simulink model "ECO_openSource"  (R2020b)
settings: Solver=FixedStepAuto  StartTime=0.0  StopTime=parECO.ref.time(end)+parECO.ref.dT  FixedStep=0.001  RelTol=1e-3  EnableMultiTasking=on
InitFcn:
  | if ~exist('parECO','var')
  |    load('parECO.mat');
  | end
  | if ~isfield(parECO,'ref')
  | 
  |    parECO.enNoise = true;
  |    parECO.enDist = true;
  |    parECO.enFB.imep = true;
  |    parECO.enFB.dpMax = true;
  |    parECO.enFB.Tevo = true;
  |    parECO.enFB.cNOx = true;
  | 
  |    parECO.ref.dT = 5;
  |    parECO.ref.imep = [  6   6   9   9   7   7 ] * 1e5
  |    parECO.ref.dpMax = [ 15   4   4   4   4   4 ] * 1e5;
  |    parECO.ref.Tevo = [  0   0   0 680   0   0 ] + 273;
  |    parECO.ref.cNOx = [100 100 100 100 100  15 ] * 1e2;
  | 
  |    parECO.ref.time  = 0 : parECO.ref.dT : parECO.ref.dT*(numel(parECO.ref.imep)-1);
  |    parECO.ref.imep  = [parECO.Reference.IMEP parECO.ref.imep(1)  parECO.ref.imep ];
  |    parECO.ref.dpMax = [parECO.Reference.dpMax parECO.ref.dpMax(1) parECO.ref.dpMax];
  |    parECO.ref.Tevo  = [parECO.Reference.Tmin parECO.ref.Tevo(1)  parECO.ref.Tevo];
  |    parECO.ref.cNOx  = [parECO.Reference.cNOx parECO.ref.cNOx(1)  parECO.ref.cNOx];
  |    parECO.ref.time  = [0 1 parECO.ref.time + parECO.ref.dT ];
  | 
  | end
undefined symbols (not defined in the file): DiscIntNeverNeededParam, parOpt, parSim
libraries: simulink x6, dspstat3 x4, dspswit3 x1, hdlsllib x1
(part 2 of 2)

== system ECO_openSource/Controller/NMPC Algorithm/Subsystem/Algorithm/Create Bounds on h_e/Scale Reference ==
  unscaled : Inport
  Sum : Sum  Inputs=|++
  offs : Constant  Value=[parECO.offsX(3); 0]
  scale : Gain  Gain=1./[parECO.scaleX(3); 1e3]
  scaled : Outport
  wires:
  unscaled/1 -> scale/1
  scale/1 -> Sum/1
  Sum/1 -> scaled/1
  offs/1 -> Sum/2

== system ECO_openSource/Controller/NMPC Algorithm/Subsystem/Algorithm/Create Bounds on h_e/Scale cNOx ==
  unscaled : Inport
  Sum : Sum  Inputs=|++
  offs : Constant  Value=0
  scale : Gain  Gain=1./1e3
  scaled : Outport
  wires:
  unscaled/1 -> scale/1
  scale/1 -> Sum/1
  Sum/1 -> scaled/1
  offs/1 -> Sum/2

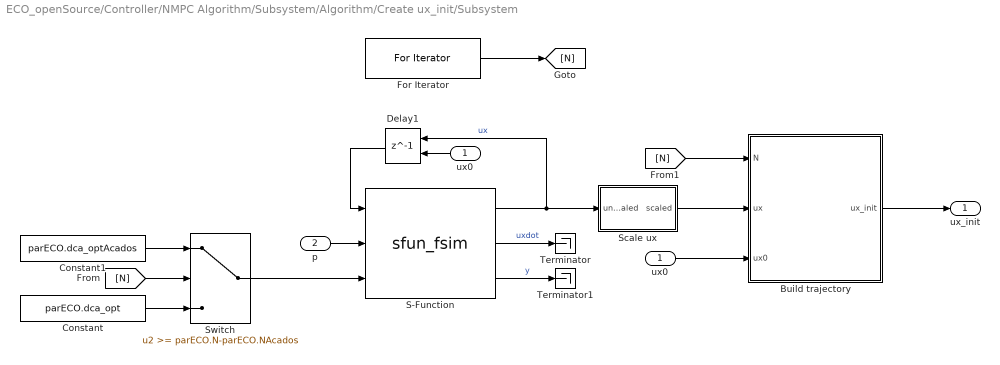
== system ECO_openSource/Controller/NMPC Algorithm/Subsystem/Algorithm/Create ux_init/Subsystem ==
  ux0 : Inport
  p : Inport  Port=2
  " ux0 " : InportShadow
  Build trajectory : Subsystem
  Constant : Constant  Value=parECO.dca_opt
  Constant1 : Constant  Value=parECO.dca_optAcados
  Delay1 : Delay  DelayLength=1  InitialConditionSource=Input port  InitialCondition=[parOpt.u0;parSim.OP.pInt;0;0]
      settings: InputPortMap=u0,p4
  For Iterator : ForIterator  ResetStates=reset  IterationLimit=parECO.N
  S-Function : S-Function  FunctionName=sfun_fsim  SFunctionDeploymentMode=off  EnableBusSupport=off
  Scale ux : Subsystem
  Switch : Switch  Threshold=parECO.N-parECO.NAcados
  Terminator : Terminator
  Terminator1 : Terminator
  ux_init : Outport
  wires:
  ux0/1 -> Delay1/2
  Delay1/1 -> S-Function/1
  " ux0 "/1 -> Build trajectory/3(ux0)
  Scale ux/1(scaled) -> Build trajectory/2(ux)
  Build trajectory/1(ux_init) -> ux_init/1
  Switch/1 -> S-Function/3
  Constant/1 -> Switch/3
  Constant1/1 -> Switch/1
  S-Function/1 -> Scale ux/1(unscaled), Delay1/1  "ux"
  S-Function/3 -> Terminator1/1  "y"
  S-Function/2 -> Terminator/1  "uxdot"
  For Iterator/1 -> [N]
  [N] -> Switch/2
  [N] -> Build trajectory/1(N)
  p/1 -> S-Function/2

== system ECO_openSource/Controller/NMPC Algorithm/Subsystem/Algorithm/Create ux_init/Unscale ux0 ==
  scaled : Inport
  Sum : Sum  Inputs=|++
  offs : Constant  Value=[parECO.offsU;parECO.offsX;parECO.offsCA]
  scale : Gain  Gain=[parECO.scaleU;parECO.scaleX;parECO.scaleCA]
  unscaled : Outport
  wires:
  offs/1 -> Sum/2
  scaled/1 -> scale/1
  scale/1 -> Sum/1
  Sum/1 -> unscaled/1

== system ECO_openSource/Controller/NMPC Algorithm/Subsystem/Algorithm/Model Simulation/Create Outputs ==
  ux : Inport
  uxdot : Inport  Port=2
  y : Inport  Port=3
  Delay : Delay  DelayLength=1
  Max : MinMax  Function=max  Inputs=2
  Mux : Mux
  Selector : Selector  InputPortWidth=10  IndexOptions=Index vector (dialog)  Indices=7  OutputSizes=1
  Selector1 : Selector  InputPortWidth=10  IndexOptions=Index vector (dialog)  Indices=5  OutputSizes=1
  Selector2 : Selector  InputPortWidth=12  IndexOptions=Index vector (dialog)  Indices=1  OutputSizes=1
  Selector3 : Selector  InputPortWidth=12  IndexOptions=Index vector (dialog)  Indices=9  OutputSizes=1
  ySim : Outport
  wires:
  ux/1 -> Selector/1
  uxdot/1 -> Selector1/1
  Selector1/1 -> Max/1
  Delay/1 -> Max/2
  Max/1 -> Delay/1, Mux/4
  Selector/1 -> Mux/1
  Mux/1 -> ySim/1
  Selector2/1 -> Mux/3
  Selector3/1 -> Mux/2
  y/1 -> Selector2/1, Selector3/1

== system ECO_openSource/Controller/NMPC Algorithm/Subsystem/Algorithm/Calculate Initial Condition/Calculate Condition at Start of Optimization/Scale ux0 ==
  unscaled : Inport
  Sum : Sum  Inputs=|+-
  offs : Constant  Value=[parECO.offsU;parECO.offsX;parECO.offsCA]
  scale : Gain  Gain=1./[parECO.scaleU;parECO.scaleX;parECO.scaleCA]
  scaled : Outport
  wires:
  offs/1 -> Sum/2
  unscaled/1 -> Sum/1
  Sum/1 -> scale/1
  scale/1 -> scaled/1

== system ECO_openSource/Controller/NMPC Algorithm/Subsystem/Algorithm/Create ux_init/Subsystem/Build trajectory ==
  N : Inport
  ux : Inport  Port=2
  ux0 : Inport  Port=3
  Delay : Delay  DelayLength=1  InitialConditionSource=Input port
      settings: InputPortMap=u0,p4
  MATLAB Function : MATLAB Function  TreatAsAtomicUnit=on
  MATLAB Function1 : MATLAB Function  TreatAsAtomicUnit=on
  Scale ux0 : Subsystem
  ux_init : Outport
  wires:
  MATLAB Function1/1(y) -> Delay/2
  Delay/1 -> MATLAB Function/3("ux_init ")
  MATLAB Function/1(ux_init) -> Delay/1, ux_init/1
  Scale ux0/1(scaled) -> MATLAB Function1/1(u)
  N/1 -> MATLAB Function/1(N)
  ux/1 -> MATLAB Function/2(ux)
  ux0/1 -> Scale ux0/1(unscaled)

== system ECO_openSource/Controller/NMPC Algorithm/Subsystem/Algorithm/Create ux_init/Subsystem/Scale ux ==
  unscaled : Inport
  Sum : Sum  Inputs=|+-
  offs : Constant  Value=[parECO.offsU;parECO.offsX;parECO.offsCA]
  scale : Gain  Gain=1./[parECO.scaleU;parECO.scaleX;parECO.scaleCA]
  scaled : Outport
  wires:
  offs/1 -> Sum/2
  unscaled/1 -> Sum/1
  Sum/1 -> scale/1
  scale/1 -> scaled/1

== system ECO_openSource/Controller/NMPC Algorithm/Subsystem/Algorithm/Create ux_init/Subsystem/Build trajectory/Scale ux0 ==
  unscaled : Inport
  Sum : Sum  Inputs=|+-
  offs : Constant  Value=[parECO.offsU;parECO.offsX;parECO.offsCA]
  scale : Gain  Gain=1./[parECO.scaleU;parECO.scaleX;parECO.scaleCA]
  scaled : Outport
  wires:
  offs/1 -> Sum/2
  unscaled/1 -> Sum/1
  Sum/1 -> scale/1
  scale/1 -> scaled/1

== matlab function ECO_openSource/Controller/Check for Reference Step/any ==
  data: u input; y output
function y = fcn(u)

y = any(u);

== matlab function ECO_openSource/Controller/NMPC Algorithm/Subsystem/Algorithm/repmat ==
  data: u input; y output; N parameter
function y = fcn(u,N)

y = repmat(u',1,N);

== matlab function ECO_openSource/Controller/NMPC Algorithm/Subsystem/Algorithm/Create Bounds on h/Extended repmat ==
  data: u input; y output; idx input size=1; parECO parameter
function y = fcn(u,idx,parECO)

% Add 2°CA to idx because of Simulink to MATLAB deviation
idx = idx+2;

% Get idxCoC in parECO.ca
idxCoC  = find(parECO.ca >= idx,1,'first');
idxCoC  = idxCoC(1); % Simulink needs to be sure idxCoC is dimension 1

% Span u over horizon and include latest CoC
y       = repmat(u',1,parECO.N);
nConstr = parECO.nConstr;

y(nConstr*idxCoC:nConstr:end) = 0;

== matlab function ECO_openSource/Controller/NMPC Algorithm/Subsystem/Algorithm/Create Bounds on h/Repmat ==
  data: u input; y output; N parameter
function y = fcn(u,N)

y = repmat(u',1,N);

== matlab function ECO_openSource/Controller/NMPC Algorithm/Subsystem/Algorithm/Create ux_init/Subsystem/Build trajectory/MATLAB Function ==
  data: N input; ux input; ux_init output; ux_init input; parECO parameter
function ux_init = fcn(N,ux,ux_init,parECO)

idx          = N * (parECO.nInputs+parECO.nStates+1) + 1 : ...
    (N+1) * (parECO.nInputs+parECO.nStates+1);
ux_init(idx)  = ux;
end

== matlab function ECO_openSource/Controller/NMPC Algorithm/Subsystem/Algorithm/Create ux_init/Subsystem/Build trajectory/MATLAB Function1 ==
  data: u input; y output; parECO parameter
function y = repMat(u,parECO)

y = repmat(u,parECO.N+1,1);

== matlab function ECO_openSource/Correct DOE for Single-Injection Operation/MATLAB Function ==
  data: u input; u output
function u = fcn(u)

% If doe < 100 mus set it to 0. Second condition to discard soe inputs
u(u < 105 & u > 50) = 0;

== matlab function ECO_openSource/Controller/NMPC Algorithm/Subsystem/Algorithm/any ==
  data: u input; y output
function y = fcn(u)

y = any(u);
